simulink model "URDF_Dynamics_Impedance"  (R2023b)
settings: Solver=VariableStepAuto  StartTime=0.0  StopTime=10.0  RelTol=1e-3
values from neighbouring files (symbols this model uses):
  Ftip = [1; 1; 1; 1; 1; 1]    [Dynamic_Test.m]    (also in Test_New_ROBOT_dynamics.m = [0; 0; 0; 0; 0; 0]; dynamic_poe_test.m = [0, 0, 0, 0, 0, 0]'; dynamic_poe_test_2.m = [0, 0, 0, 0, 0, 0]'; dynamic_poe_test_3.m = [0, 0, 0, 0, 0, 0]')
  g_vec = [0; 0; -9.81]    [Test_New_ROBOT_dynamics.m]    (also in dynamic_poe_test.m = [0, 0, -9.81]'; dynamic_poe_test_2.m = [0, 0, 9.81]'; dynamic_poe_test_3.m = [0, 0, -9.81]')
  Glist = cat(3, G1, G2, G3)    [Dynamic_Test.m]    (also in Test_New_ROBOT_dynamics.m = zeros(6, 6, 6); dynamic_poe_test.m = cat(3, G1, G2, G3, G4, G5, G6); dynamic_poe_test_2.m = cat(3, G1, G2, G3, G4, G5, G6); dynamic_poe_test_3.m = cat(3, G1, G2, G3, G4, G5, G6))
  m = 0.1062    [Test_New_ROBOT_dynamics.m]
  Mlist = zeros(4,4,n+1)    [DH_to_Mlist.m]    (also in DH_to_Mlist_Test.m = DH_to_Mlist(DH); Dynamic_Test.m = cat(3, M01, M12, M23, M34); ForwardPOE_Test.m = cat(3, M1, M2, M3, M4, M5, M6, M7); ForwardPOE_Test_2.m = cat(3, M1, M2, M3, M4, M5, M6, M7))
  Slist = [1, 0, 0 ... (first row only)    [Dynamic_Test.m]    (also in ForwardPOE_Test.m = [S1, S2, S3, S4, S5, S6]; ForwardPOE_Test_2.m = [S1, S2, S3, S4, S5, S6]; Make_Slist.m = zeros(6, num_joints); Make_Slist_2.m = zeros(6, num_joints))
undefined symbols (not defined in the file or in its folder): X, Y, Z
libraries: sm_lib x125, nesl_utility x43, simulink x8, robotcorelib x2, simulink_extras x1
(part 3 of 3)

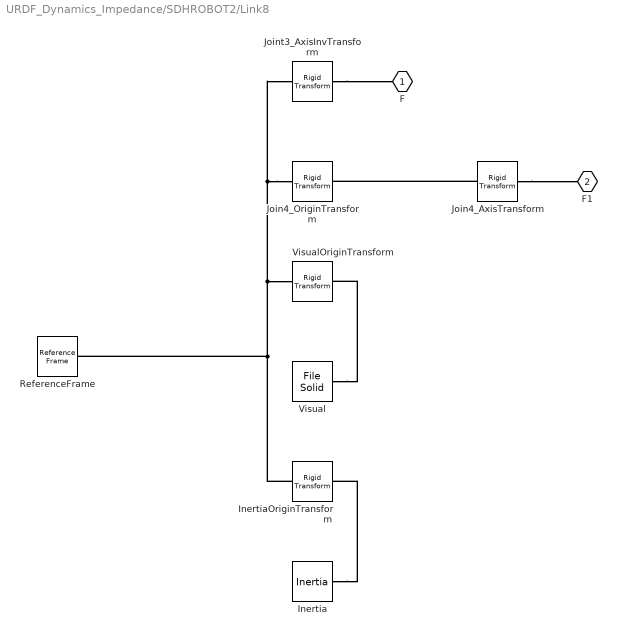
== system URDF_Dynamics_Impedance/SDHROBOT2/Link8 ==
  Inertia : sm_lib/Body Elements/Inertia  InertiaType=Custom  Mass=0.97684  MassUnits=kg  CenterOfMass=[0, 0, 0]  CenterOfMassUnits=m  MomentsOfInertia=[0.0002136, 0.00045138, 0.00033322]  MomentsOfInertiaUnits=kg*m^2  ProductsOfInertia=[2.6957e-06, 7.4844e-05, -5.0865e-06]  ProductsOfInertiaUnits=kg*m^2  GraphicType=None  MarkerShape=Inertia  MarkerSize=20  GraphicVisPropType=SimpleVisualProperties  GraphicDiffuseColor=[0.5 0.5 0.5]  GraphicSpecularColor=[0.5 0.5 0.5 1.0]  GraphicAmbientColor=[0.15 0.15 0.15 1.0]  GraphicEmissiveColor=[0.0 0.0 0.0 1.0]  GraphicShininess=75  GraphicOpacity=1.0
  InertiaOriginTransform : sm_lib/Frames and Transforms/Rigid Transform  TranslationMethod=Cartesian  TranslationStandardOffset=0  TranslationStandardOffsetUnits=m  TranslationStandardAxis=+Z  TranslationCartesianOffset=[0.045234, -0.014686, 0.0040411]  TranslationCartesianOffsetUnits=m  TranslationROffset=0  TranslationROffsetUnits=m  TranslationZOffset=0  TranslationZOffsetUnits=m  TranslationThetaOffset=0  TranslationThetaOffsetUnits=deg  RotationMethod=RotationSequence  RotationAngleUnits=deg  RotationStandardAxis=+Z  RotationAngle=0.0  RotationArbitraryAxis=[0 0 1]  FollAlignAxisA=+X  BaseAlignAxisA=+Y  FollAlignAxisB=+Y  BaseAlignAxisB=+Z  RotationSequenceAxes=BaseAxes  RotationSequence=XYZ  RotationSequenceAngles=[0, 0, 0]  RotationSequenceAnglesUnits=rad  RotationMatrix=[1 0 0; 0 1 0; 0 0 1]  Quaternion=[1 0 0 0]
  Join4_AxisTransform : sm_lib/Frames and Transforms/Rigid Transform  TranslationMethod=Cartesian  TranslationStandardOffset=0  TranslationStandardOffsetUnits=m  TranslationStandardAxis=+Z  TranslationCartesianOffset=[0, 0, 0]  TranslationCartesianOffsetUnits=m  TranslationROffset=0  TranslationROffsetUnits=m  TranslationZOffset=0  TranslationZOffsetUnits=m  TranslationThetaOffset=0  TranslationThetaOffsetUnits=deg  RotationMethod=ArbitraryAxis  RotationAngleUnits=rad  RotationStandardAxis=+Z  RotationAngle=0  RotationArbitraryAxis=[1, 0, 0]  FollAlignAxisA=+X  BaseAlignAxisA=+Y  FollAlignAxisB=+Y  BaseAlignAxisB=+Z  RotationSequenceAxes=FollowerAxes  RotationSequence=XYX  RotationSequenceAngles=[0 0 0]  RotationSequenceAnglesUnits=deg  RotationMatrix=[1 0 0; 0 1 0; 0 0 1]  Quaternion=[1 0 0 0]
  Join4_OriginTransform : sm_lib/Frames and Transforms/Rigid Transform  TranslationMethod=Cartesian  TranslationStandardOffset=0  TranslationStandardOffsetUnits=m  TranslationStandardAxis=+Z  TranslationCartesianOffset=[0.052, 0, 0]  TranslationCartesianOffsetUnits=m  TranslationROffset=0  TranslationROffsetUnits=m  TranslationZOffset=0  TranslationZOffsetUnits=m  TranslationThetaOffset=0  TranslationThetaOffsetUnits=deg  RotationMethod=RotationSequence  RotationAngleUnits=deg  RotationStandardAxis=+Z  RotationAngle=0.0  RotationArbitraryAxis=[0 0 1]  FollAlignAxisA=+X  BaseAlignAxisA=+Y  FollAlignAxisB=+Y  BaseAlignAxisB=+Z  RotationSequenceAxes=BaseAxes  RotationSequence=XYZ  RotationSequenceAngles=[-1.5708, 0, 0]  RotationSequenceAnglesUnits=rad  RotationMatrix=[1 0 0; 0 1 0; 0 0 1]  Quaternion=[1 0 0 0]
  Joint3_AxisInvTransform : sm_lib/Frames and Transforms/Rigid Transform  TranslationMethod=Cartesian  TranslationStandardOffset=0  TranslationStandardOffsetUnits=m  TranslationStandardAxis=+Z  TranslationCartesianOffset=[0, 0, 0]  TranslationCartesianOffsetUnits=m  TranslationROffset=0  TranslationROffsetUnits=m  TranslationZOffset=0  TranslationZOffsetUnits=m  TranslationThetaOffset=0  TranslationThetaOffsetUnits=deg  RotationMethod=ArbitraryAxis  RotationAngleUnits=rad  RotationStandardAxis=+Z  RotationAngle=0  RotationArbitraryAxis=[1, 0, 0]  FollAlignAxisA=+X  BaseAlignAxisA=+Y  FollAlignAxisB=+Y  BaseAlignAxisB=+Z  RotationSequenceAxes=FollowerAxes  RotationSequence=XYX  RotationSequenceAngles=[0 0 0]  RotationSequenceAnglesUnits=deg  RotationMatrix=[1 0 0; 0 1 0; 0 0 1]  Quaternion=[1 0 0 0]
  ReferenceFrame : sm_lib/Frames and Transforms/Reference Frame
  Visual : sm_lib/Body Elements/File Solid  ExtGeomFileName=URDFDummy4/meshes/Link3.STL  UnitType=Custom  ExtGeomFileUnits=m  StepReaderType=HEX  ExportConvexHullGeometry=off  InertiaType=Custom  Mass=0  MassUnits=kg  CenterOfMass=[0, 0, 0]  CenterOfMassUnits=m  MomentsOfInertia=[0, 0, 0]  MomentsOfInertiaUnits=kg*m^2  ProductsOfInertia=[0, 0, 0]  ProductsOfInertiaUnits=kg*m^2  BasedOnType=DensityFromFile  Density=1000  DensityUnits=kg/m^3  DoExposeReferenceFrame=on  SerializedFrames=<Frames/>  GraphicType=FromGeometry  MarkerShape=Sphere  MarkerSize=10  GraphicVisPropType=SimpleVisualProperties  GraphicDiffuseColor=[0.7529400000000001, 0.7529400000000001, 0.7529400000000001]  GraphicSpecularColor=[0.5 0.5 0.5 1.0]  GraphicAmbientColor=[0.15 0.15 0.15 1.0]  GraphicEmissiveColor=[0.0 0.0 0.0 1.0]  GraphicShininess=75  GraphicOpacity=1
  VisualOriginTransform : sm_lib/Frames and Transforms/Rigid Transform  TranslationMethod=Cartesian  TranslationStandardOffset=0  TranslationStandardOffsetUnits=m  TranslationStandardAxis=+Z  TranslationCartesianOffset=[0, 0, 0]  TranslationCartesianOffsetUnits=m  TranslationROffset=0  TranslationROffsetUnits=m  TranslationZOffset=0  TranslationZOffsetUnits=m  TranslationThetaOffset=0  TranslationThetaOffsetUnits=deg  RotationMethod=RotationSequence  RotationAngleUnits=deg  RotationStandardAxis=+Z  RotationAngle=0.0  RotationArbitraryAxis=[0 0 1]  FollAlignAxisA=+X  BaseAlignAxisA=+Y  FollAlignAxisB=+Y  BaseAlignAxisB=+Z  RotationSequenceAxes=BaseAxes  RotationSequence=XYZ  RotationSequenceAngles=[0, 0, 0]  RotationSequenceAnglesUnits=rad  RotationMatrix=[1 0 0; 0 1 0; 0 0 1]  Quaternion=[1 0 0 0]
  F : PMIOPort  Side=Left
  F1 : PMIOPort  Port=2  Side=Right
  connections:
  Inertia/RConn1 -- InertiaOriginTransform/RConn1
  Join4_AxisTransform/RConn1 -- F1/RConn1
  Join4_AxisTransform/LConn1 -- Join4_OriginTransform/RConn1
  Joint3_AxisInvTransform/RConn1 -- F/RConn1
  Join4_OriginTransform/LConn1 -- Joint3_AxisInvTransform/LConn1 -- InertiaOriginTransform/LConn1 -- ReferenceFrame/RConn1 -- VisualOriginTransform/LConn1
  Visual/RConn1 -- VisualOriginTransform/RConn1

== system URDF_Dynamics_Impedance/SDHROBOT2/Link9 ==
  Inertia : sm_lib/Body Elements/Inertia  InertiaType=Custom  Mass=0.78186  MassUnits=kg  CenterOfMass=[0, 0, 0]  CenterOfMassUnits=m  MomentsOfInertia=[0.00031278, 0.00036955, 0.00010046]  MomentsOfInertiaUnits=kg*m^2  ProductsOfInertia=[-2.2564e-05, -1.1305e-07, 2.8892e-09]  ProductsOfInertiaUnits=kg*m^2  GraphicType=None  MarkerShape=Inertia  MarkerSize=20  GraphicVisPropType=SimpleVisualProperties  GraphicDiffuseColor=[0.5 0.5 0.5]  GraphicSpecularColor=[0.5 0.5 0.5 1.0]  GraphicAmbientColor=[0.15 0.15 0.15 1.0]  GraphicEmissiveColor=[0.0 0.0 0.0 1.0]  GraphicShininess=75  GraphicOpacity=1.0
  InertiaOriginTransform : sm_lib/Frames and Transforms/Rigid Transform  TranslationMethod=Cartesian  TranslationStandardOffset=0  TranslationStandardOffsetUnits=m  TranslationStandardAxis=+Z  TranslationCartesianOffset=[3.1941e-05, -0.001882, 0.07442500000000001]  TranslationCartesianOffsetUnits=m  TranslationROffset=0  TranslationROffsetUnits=m  TranslationZOffset=0  TranslationZOffsetUnits=m  TranslationThetaOffset=0  TranslationThetaOffsetUnits=deg  RotationMethod=RotationSequence  RotationAngleUnits=deg  RotationStandardAxis=+Z  RotationAngle=0.0  RotationArbitraryAxis=[0 0 1]  FollAlignAxisA=+X  BaseAlignAxisA=+Y  FollAlignAxisB=+Y  BaseAlignAxisB=+Z  RotationSequenceAxes=BaseAxes  RotationSequence=XYZ  RotationSequenceAngles=[0, 0, 0]  RotationSequenceAnglesUnits=rad  RotationMatrix=[1 0 0; 0 1 0; 0 0 1]  Quaternion=[1 0 0 0]
  Join4_AxisInvTransform : sm_lib/Frames and Transforms/Rigid Transform  TranslationMethod=Cartesian  TranslationStandardOffset=0  TranslationStandardOffsetUnits=m  TranslationStandardAxis=+Z  TranslationCartesianOffset=[0, 0, 0]  TranslationCartesianOffsetUnits=m  TranslationROffset=0  TranslationROffsetUnits=m  TranslationZOffset=0  TranslationZOffsetUnits=m  TranslationThetaOffset=0  TranslationThetaOffsetUnits=deg  RotationMethod=ArbitraryAxis  RotationAngleUnits=rad  RotationStandardAxis=+Z  RotationAngle=0  RotationArbitraryAxis=[1, 0, 0]  FollAlignAxisA=+X  BaseAlignAxisA=+Y  FollAlignAxisB=+Y  BaseAlignAxisB=+Z  RotationSequenceAxes=FollowerAxes  RotationSequence=XYX  RotationSequenceAngles=[0 0 0]  RotationSequenceAnglesUnits=deg  RotationMatrix=[1 0 0; 0 1 0; 0 0 1]  Quaternion=[1 0 0 0]
  Joint5_AxisTransform : sm_lib/Frames and Transforms/Rigid Transform  TranslationMethod=Cartesian  TranslationStandardOffset=0  TranslationStandardOffsetUnits=m  TranslationStandardAxis=+Z  TranslationCartesianOffset=[0, 0, 0]  TranslationCartesianOffsetUnits=m  TranslationROffset=0  TranslationROffsetUnits=m  TranslationZOffset=0  TranslationZOffsetUnits=m  TranslationThetaOffset=0  TranslationThetaOffsetUnits=deg  RotationMethod=ArbitraryAxis  RotationAngleUnits=rad  RotationStandardAxis=+Z  RotationAngle=0  RotationArbitraryAxis=[1, 0, 0]  FollAlignAxisA=+X  BaseAlignAxisA=+Y  FollAlignAxisB=+Y  BaseAlignAxisB=+Z  RotationSequenceAxes=FollowerAxes  RotationSequence=XYX  RotationSequenceAngles=[0 0 0]  RotationSequenceAnglesUnits=deg  RotationMatrix=[1 0 0; 0 1 0; 0 0 1]  Quaternion=[1 0 0 0]
  Joint5_OriginTransform : sm_lib/Frames and Transforms/Rigid Transform  TranslationMethod=Cartesian  TranslationStandardOffset=0  TranslationStandardOffsetUnits=m  TranslationStandardAxis=+Z  TranslationCartesianOffset=[0, 0, 0.117]  TranslationCartesianOffsetUnits=m  TranslationROffset=0  TranslationROffsetUnits=m  TranslationZOffset=0  TranslationZOffsetUnits=m  TranslationThetaOffset=0  TranslationThetaOffsetUnits=deg  RotationMethod=RotationSequence  RotationAngleUnits=deg  RotationStandardAxis=+Z  RotationAngle=0.0  RotationArbitraryAxis=[0 0 1]  FollAlignAxisA=+X  BaseAlignAxisA=+Y  FollAlignAxisB=+Y  BaseAlignAxisB=+Z  RotationSequenceAxes=BaseAxes  RotationSequence=XYZ  RotationSequenceAngles=[1.5708, 0, 0]  RotationSequenceAnglesUnits=rad  RotationMatrix=[1 0 0; 0 1 0; 0 0 1]  Quaternion=[1 0 0 0]
  ReferenceFrame : sm_lib/Frames and Transforms/Reference Frame
  Visual : sm_lib/Body Elements/File Solid  ExtGeomFileName=URDFDummy4/meshes/Link4.STL  UnitType=Custom  ExtGeomFileUnits=m  StepReaderType=HEX  ExportConvexHullGeometry=off  InertiaType=Custom  Mass=0  MassUnits=kg  CenterOfMass=[0, 0, 0]  CenterOfMassUnits=m  MomentsOfInertia=[0, 0, 0]  MomentsOfInertiaUnits=kg*m^2  ProductsOfInertia=[0, 0, 0]  ProductsOfInertiaUnits=kg*m^2  BasedOnType=DensityFromFile  Density=1000  DensityUnits=kg/m^3  DoExposeReferenceFrame=on  SerializedFrames=<Frames/>  GraphicType=FromGeometry  MarkerShape=Sphere  MarkerSize=10  GraphicVisPropType=SimpleVisualProperties  GraphicDiffuseColor=[0.7529400000000001, 0.7529400000000001, 0.7529400000000001]  GraphicSpecularColor=[0.5 0.5 0.5 1.0]  GraphicAmbientColor=[0.15 0.15 0.15 1.0]  GraphicEmissiveColor=[0.0 0.0 0.0 1.0]  GraphicShininess=75  GraphicOpacity=1
  VisualOriginTransform : sm_lib/Frames and Transforms/Rigid Transform  TranslationMethod=Cartesian  TranslationStandardOffset=0  TranslationStandardOffsetUnits=m  TranslationStandardAxis=+Z  TranslationCartesianOffset=[0, 0, 0]  TranslationCartesianOffsetUnits=m  TranslationROffset=0  TranslationROffsetUnits=m  TranslationZOffset=0  TranslationZOffsetUnits=m  TranslationThetaOffset=0  TranslationThetaOffsetUnits=deg  RotationMethod=RotationSequence  RotationAngleUnits=deg  RotationStandardAxis=+Z  RotationAngle=0.0  RotationArbitraryAxis=[0 0 1]  FollAlignAxisA=+X  BaseAlignAxisA=+Y  FollAlignAxisB=+Y  BaseAlignAxisB=+Z  RotationSequenceAxes=BaseAxes  RotationSequence=XYZ  RotationSequenceAngles=[0, 0, 0]  RotationSequenceAnglesUnits=rad  RotationMatrix=[1 0 0; 0 1 0; 0 0 1]  Quaternion=[1 0 0 0]
  F : PMIOPort  Side=Left
  F1 : PMIOPort  Port=2  Side=Right
  connections:
  Inertia/RConn1 -- InertiaOriginTransform/RConn1
  Join4_AxisInvTransform/RConn1 -- F/RConn1
  Joint5_AxisTransform/RConn1 -- F1/RConn1
  Joint5_AxisTransform/LConn1 -- Joint5_OriginTransform/RConn1
  Join4_AxisInvTransform/LConn1 -- InertiaOriginTransform/LConn1 -- Joint5_OriginTransform/LConn1 -- ReferenceFrame/RConn1 -- VisualOriginTransform/LConn1
  Visual/RConn1 -- VisualOriginTransform/RConn1

== matlab function URDF_Dynamics_Impedance/MATLAB Function1 ==
  data: q_desired input; tau output; dq_desired input; ddq_desired input; q input; dq input; ddq input
function tau = JointImpedanceControl(q_desired, dq_desired, ddq_desired, q, dq, ddq)
% JOINTIMPEDANCECONTROL 关节空间阻抗控制器
%
% 适用于:
%   1. 定点阻抗控制: dq_desired = 0, ddq_desired = 0
%   2. 轨迹跟踪阻抗控制: 输入时变轨迹
%
% 控制方程:
%   tau = M_d * (ddq_d - ddq) + B_d * (dq_d - dq) + K_d * (q_d - q)

    %% 关节数
    n = length(q);
    
    %% 阻抗参数 (根据应用调整)
    % -------------------------------------------------
    % 定点阻抗: K较小 -> 柔顺性好, 适合接触任务
    % 轨迹跟踪: K较大 -> 跟踪精度高
    % -------------------------------------------------
    
    % 刚度 [N·m/rad]
    K = [2000; 2000; 1500; 1500; 1000; 500; 200];
    K = K(1:n);
    
    % 阻尼 [N·m·s/rad] - 临界阻尼系数
    B = 2 * sqrt(K);
    
    % 惯量 [kg·m²]
    M = ones(n, 1);
    
    %% 误差计算
    e_q   = q_desired - q;
    e_dq  = dq_desired - dq;
    e_ddq = ddq_desired - ddq;
    
    %% 阻抗控制力矩
    tau = M .* e_ddq + B .* e_dq + K .* e_q;

end

== matlab function URDF_Dynamics_Impedance/MATLAB Function ==
  data: thetas input; tau output; dthetas input; ddthetas input; g input; Ftip input; Mlist input; Glist input; Slist input
function tau = InverseDynamics(thetas, dthetas, ddthetas, g, Ftip, Mlist, Glist, Slist)
% INVERSEDYNAMICS 计算串联机械臂的逆动力学
%
% 输入:
%   thetas:   n x 1 关节角
%   dthetas:  n x 1 关节角速度
%   ddthetas: n x 1 关节角加速度
%   g:        3 x 1 重力向量 (例如 [0; 0; -9.81])
%   Ftip:     6 x 1 末端受力 (空间力 Wrench: [力矩; 力])
%   Mlist:    4 x 4 x (n+1) 初始位姿列表 (M_0_1, M_1_2, ... M_n_end)
%   Glist:    6 x 6 x n 空间惯量矩阵列表
%   Slist:    6 x n 空间螺旋轴列表
%
% 输出:
%   tau:      n x 1 关节力矩向量

    % 1. 参数提取与初始化
    n = size(thetas, 1);
    
    % 初始化 M_i-1_i (当前关节相对上一关节的变换矩阵)
    % 注意：Mlist(:,:,i) 存储的是 M_{i-1, i}
    Mi = eye(4); 
    
    % 将空间螺旋轴 Slist 转换为体螺旋轴 Blist (Ai)
    % 这里的逻辑是：Ai = Ad_inv(M_0_i) * Si
    Alist = zeros(6, n);
    M_0_i = eye(4); % 累积变换 M_0_1 * M_1_2 ...
    
    for i = 1:n
        M_0_i = M_0_i * Mlist(:,:,i);     % 计算基座到当前连杆i的零位变换
        Alist(:, i) = Adjoint(TransInv(M_0_i)) * Slist(:, i); 
    end

    % 2. 前向递推 (Forward Iteration): 计算速度 V 和 加速度 Vdot
    % Vlist, VdotList 存储在体坐标系下的值
    Vlist = zeros(6, n+1);    % V0 ... Vn
    VdotList = zeros(6, n+1); % Vdot0 ... Vdotn
    
    % 初始化基座状态 (V0=0, Vdot0用重力模拟)
    % Vdot0 设置为重力的反向加速度，等效于重力作用
    % g = [gx, gy, gz], Vdot0 = [0;0;0; -g] 因为 Vdot 是 [ang_acc; lin_acc]
    VdotList(:, 1) = [0; 0; 0; -g]; 
    
    % 保存各连杆间的变换矩阵 T_i_iminus1 (T_{i, i-1}) 供后向使用
    T_list = zeros(4, 4, n+1); 

    for i = 1:n
        % 计算 T_{i-1, i} = M_{i-1, i} * exp( [Ai] * theta )
        % 但我们需要 T_{i, i-1} = T_{i-1, i}^-1
        % T_{i, i-1} = exp( -[Ai] * theta ) * M_{i-1, i}^-1
        
        M_i_iminus1 = TransInv(Mlist(:,:,i));
        T_i_iminus1 = MatrixExp6(VecTose3(Alist(:,i) * -thetas(i))) * M_i_iminus1;
        
        T_list(:,:,i) = T_i_iminus1; % 存起来
        
        % 速度传递: V_i = Ad_T_i_i-1 * V_i-1 + A_i * dtheta_i
        Ad_T = Adjoint(T_i_iminus1);
        Vlist(:, i+1) = Ad_T * Vlist(:, i) + Alist(:, i) * dthetas(i);
        
        % 加速度传递: Vdot_i = Ad_T * Vdot_i-1 + ad_Vi * (Ai*dtheta) + Ai*ddtheta
        % ad_Vi * Ai*dtheta 这一项就是科里奥利力项 (Lie Bracket)
        ad_V = ad(Vlist(:, i+1));
        term_coriolis = ad_V * (Alist(:, i) * dthetas(i));
        
        VdotList(:, i+1) = Ad_T * VdotList(:, i) + term_coriolis + Alist(:, i) * ddthetas(i);
    end

    % 3. 后向递推 (Backward Iteration): 计算力 F 和 力矩 tau
    tau = zeros(n, 1);
    
    % 处理末端受力: Ftip 是末端施加给环境的力，反作用力是 -Ftip? 
    % 通常 Ftip 定义为环境施加给末端的力。如果是这样直接用。
    % 这里我们假设输入的 Ftip 是“末端Link受到的外力”。
    % 我们需要把它转换到 Link n 的坐标系。
    % Mlist(:,:,n+1) 是 Link_n 到 EndEffector 的变换 M_n_end
    % 假设 Ftip 是在 EndEffector 坐标系定义的，需变换回 Link n
    M_n_end = Mlist(:,:,n+1);
    F_next = Adjoint(TransInv(M_n_end))' * Ftip; 
    
    for i = n:-1:1
        Gi = Glist(:,:,i);
        Vi = Vlist(:, i+1);
        Vdoti = VdotList(:, i+1);
        
        % 牛顿-欧拉方程 (空间形式):
        % F_i = G * Vdot - ad_V' * (G * V) + Ad_T_next_curr' * F_next
        
        % 惯性项 + 陀螺力矩项
        F_inertial = Gi * Vdoti - ad(Vi)' * (Gi * Vi);
        
        % 加上来自下一个连杆传递回来的力
        % 如果 i < n, 需要变换 F_{i+1} 到 F_i
        if i < n
             % T_{i+1, i} 来自前面的 T_list
             % 前面存的是 T_{i, i-1} (第i个), 所以 T_{i+1, i} 是 T_list(:,:,i+1)
             T_next_curr = T_list(:,:,i+1);
             F_from_next = Adjoint(T_next_curr)' * F_next;
        else
             % 如果是最后一个连杆，F_from_next 已经是我们上面算的 Ftip 转换后的
             F_from_next = F_next;
        end
        
        Fi = F_inertial + F_from_next;
        
        % 提取关节力矩: 投影到关节轴 Ai 上
        tau(i) = Fi' * Alist(:, i);
        
        % 更新 F_next 给下一次循环
        F_next = Fi;
    end
end

%% ============ 依赖的辅助函数 (若已有库可删除) ============

function AdT = Adjoint(T)
    [R, p] = TransToRp(T);
    AdT = [R, zeros(3); VecToso3(p)*R, R];
end

function se3mat = VecTose3(V)
    % V = [w; v]
    w = V(1:3); v = V(4:6);
    se3mat = [VecToso3(w), v; 0 0 0 0];
end

function so3mat = VecToso3(omg)
    so3mat = [0, -omg(3), omg(2);
              omg(3), 0, -omg(1);
             -omg(2), omg(1), 0];
end

function adV = ad(V)
    w = V(1:3); v = V(4:6);
    adV = [VecToso3(w), zeros(3); VecToso3(v), VecToso3(w)];
end

function invT = TransInv(T)
    [R, p] = TransToRp(T);
    invT = [R', -R'*p; 0 0 0 1];
end

function [R, p] = TransToRp(T)
    R = T(1:3, 1:3);
    p = T(1:3, 4);
end

function T = MatrixExp6(se3mat)
    % 简化的指数映射 (罗德里格斯公式)
    omgtheta = so3ToVec(se3mat(1:3, 1:3));
    if norm(omgtheta) < 1e-6
        T = [eye(3), se3mat(1:3, 4); 0 0 0 1];
    else
        theta = norm(omgtheta);
        omg = omgtheta / theta;
        omgmat = se3mat(1:3, 1:3) / theta;
        R = eye(3) + sin(theta)*omgmat + (1-cos(theta))*(omgmat^2);
        v = se3mat(1:3, 4) / theta;
        p = (eye(3)*theta + (1-cos(theta))*omgmat + (theta-sin(theta))*(omgmat^2)) * v;
        T = [R, p; 0 0 0 1];
    end
end

function omg = so3ToVec(so3mat)
    omg = [so3mat(3,2); so3mat(1,3); so3mat(2,1)];
end

== matlab function URDF_Dynamics_Impedance/MATLAB Function2 ==
  data: thetas input; tau output; dthetas input; ddthetas input; g input; Ftip input; Mlist input; Glist input; Slist input
function tau = InverseDynamics(thetas, dthetas, ddthetas, g, Ftip, Mlist, Glist, Slist)
% INVERSEDYNAMICS 计算串联机械臂的逆动力学
%
% 输入:
%   thetas:   n x 1 关节角
%   dthetas:  n x 1 关节角速度
%   ddthetas: n x 1 关节角加速度
%   g:        3 x 1 重力向量 (例如 [0; 0; -9.81])
%   Ftip:     6 x 1 末端受力 (空间力 Wrench: [力矩; 力])
%   Mlist:    4 x 4 x (n+1) 初始位姿列表 (M_0_1, M_1_2, ... M_n_end)
%   Glist:    6 x 6 x n 空间惯量矩阵列表
%   Slist:    6 x n 空间螺旋轴列表
%
% 输出:
%   tau:      n x 1 关节力矩向量

    % 1. 参数提取与初始化
    n = size(thetas, 1);
    
    % 初始化 M_i-1_i (当前关节相对上一关节的变换矩阵)
    % 注意：Mlist(:,:,i) 存储的是 M_{i-1, i}
    Mi = eye(4); 
    
    % 将空间螺旋轴 Slist 转换为体螺旋轴 Blist (Ai)
    % 这里的逻辑是：Ai = Ad_inv(M_0_i) * Si
    Alist = zeros(6, n);
    M_0_i = eye(4); % 累积变换 M_0_1 * M_1_2 ...
    
    for i = 1:n
        M_0_i = M_0_i * Mlist(:,:,i);     % 计算基座到当前连杆i的零位变换
        Alist(:, i) = Adjoint(TransInv(M_0_i)) * Slist(:, i); 
    end

    % 2. 前向递推 (Forward Iteration): 计算速度 V 和 加速度 Vdot
    % Vlist, VdotList 存储在体坐标系下的值
    Vlist = zeros(6, n+1);    % V0 ... Vn
    VdotList = zeros(6, n+1); % Vdot0 ... Vdotn
    
    % 初始化基座状态 (V0=0, Vdot0用重力模拟)
    % Vdot0 设置为重力的反向加速度，等效于重力作用
    % g = [gx, gy, gz], Vdot0 = [0;0;0; -g] 因为 Vdot 是 [ang_acc; lin_acc]
    VdotList(:, 1) = [0; 0; 0; -g]; 
    
    % 保存各连杆间的变换矩阵 T_i_iminus1 (T_{i, i-1}) 供后向使用
    T_list = zeros(4, 4, n+1); 

    for i = 1:n
        % 计算 T_{i-1, i} = M_{i-1, i} * exp( [Ai] * theta )
        % 但我们需要 T_{i, i-1} = T_{i-1, i}^-1
        % T_{i, i-1} = exp( -[Ai] * theta ) * M_{i-1, i}^-1
        
        M_i_iminus1 = TransInv(Mlist(:,:,i));
        T_i_iminus1 = MatrixExp6(VecTose3(Alist(:,i) * -thetas(i))) * M_i_iminus1;
        
        T_list(:,:,i) = T_i_iminus1; % 存起来
        
        % 速度传递: V_i = Ad_T_i_i-1 * V_i-1 + A_i * dtheta_i
        Ad_T = Adjoint(T_i_iminus1);
        Vlist(:, i+1) = Ad_T * Vlist(:, i) + Alist(:, i) * dthetas(i);
        
        % 加速度传递: Vdot_i = Ad_T * Vdot_i-1 + ad_Vi * (Ai*dtheta) + Ai*ddtheta
        % ad_Vi * Ai*dtheta 这一项就是科里奥利力项 (Lie Bracket)
        ad_V = ad(Vlist(:, i+1));
        term_coriolis = ad_V * (Alist(:, i) * dthetas(i));
        
        VdotList(:, i+1) = Ad_T * VdotList(:, i) + term_coriolis + Alist(:, i) * ddthetas(i);
    end

    % 3. 后向递推 (Backward Iteration): 计算力 F 和 力矩 tau
    tau = zeros(n, 1);
    
    % 处理末端受力: Ftip 是末端施加给环境的力，反作用力是 -Ftip? 
    % 通常 Ftip 定义为环境施加给末端的力。如果是这样直接用。
    % 这里我们假设输入的 Ftip 是“末端Link受到的外力”。
    % 我们需要把它转换到 Link n 的坐标系。
    % Mlist(:,:,n+1) 是 Link_n 到 EndEffector 的变换 M_n_end
    % 假设 Ftip 是在 EndEffector 坐标系定义的，需变换回 Link n
    M_n_end = Mlist(:,:,n+1);
    F_next = Adjoint(TransInv(M_n_end))' * Ftip; 
    
    for i = n:-1:1
        Gi = Glist(:,:,i);
        Vi = Vlist(:, i+1);
        Vdoti = VdotList(:, i+1);
        
        % 牛顿-欧拉方程 (空间形式):
        % F_i = G * Vdot - ad_V' * (G * V) + Ad_T_next_curr' * F_next
        
        % 惯性项 + 陀螺力矩项
        F_inertial = Gi * Vdoti - ad(Vi)' * (Gi * Vi);
        
        % 加上来自下一个连杆传递回来的力
        % 如果 i < n, 需要变换 F_{i+1} 到 F_i
        if i < n
             % T_{i+1, i} 来自前面的 T_list
             % 前面存的是 T_{i, i-1} (第i个), 所以 T_{i+1, i} 是 T_list(:,:,i+1)
             T_next_curr = T_list(:,:,i+1);
             F_from_next = Adjoint(T_next_curr)' * F_next;
        else
             % 如果是最后一个连杆，F_from_next 已经是我们上面算的 Ftip 转换后的
             F_from_next = F_next;
        end
        
        Fi = F_inertial + F_from_next;
        
        % 提取关节力矩: 投影到关节轴 Ai 上
        tau(i) = Fi' * Alist(:, i);
        
        % 更新 F_next 给下一次循环
        F_next = Fi;
    end
end

%% ============ 依赖的辅助函数 (若已有库可删除) ============

function AdT = Adjoint(T)
    [R, p] = TransToRp(T);
    AdT = [R, zeros(3); VecToso3(p)*R, R];
end

function se3mat = VecTose3(V)
    % V = [w; v]
    w = V(1:3); v = V(4:6);
    se3mat = [VecToso3(w), v; 0 0 0 0];
end

function so3mat = VecToso3(omg)
    so3mat = [0, -omg(3), omg(2);
              omg(3), 0, -omg(1);
             -omg(2), omg(1), 0];
end

function adV = ad(V)
    w = V(1:3); v = V(4:6);
    adV = [VecToso3(w), zeros(3); VecToso3(v), VecToso3(w)];
end

function invT = TransInv(T)
    [R, p] = TransToRp(T);
    invT = [R', -R'*p; 0 0 0 1];
end

function [R, p] = TransToRp(T)
    R = T(1:3, 1:3);
    p = T(1:3, 4);
end

function T = MatrixExp6(se3mat)
    % 简化的指数映射 (罗德里格斯公式)
    omgtheta = so3ToVec(se3mat(1:3, 1:3));
    if norm(omgtheta) < 1e-6
        T = [eye(3), se3mat(1:3, 4); 0 0 0 1];
    else
        theta = norm(omgtheta);
        omg = omgtheta / theta;
        omgmat = se3mat(1:3, 1:3) / theta;
        R = eye(3) + sin(theta)*omgmat + (1-cos(theta))*(omgmat^2);
        v = se3mat(1:3, 4) / theta;
        p = (eye(3)*theta + (1-cos(theta))*omgmat + (theta-sin(theta))*(omgmat^2)) * v;
        T = [R, p; 0 0 0 1];
    end
end

function omg = so3ToVec(so3mat)
    omg = [so3mat(3,2); so3mat(1,3); so3mat(2,1)];
end
